simulink model "Ej_parcial_2019_sim"  (R2018a)
settings: Solver=FixedStepAuto  StartTime=0.0  StopTime=20  FixedStep=1e-5  RelTol=1e-3
values from neighbouring files (symbols this model uses):
  Ts = 0.0001    [Bolita_2.m]    (also in Ej_parcial_2019.m = 0.1; les_boles_de_les_pibardes.m = 0.01)
undefined symbols (not defined in the file or in its folder): DiscIntNeverNeededParam
settings Model: Creator=Guido L  LastModifiedBy=Guido L

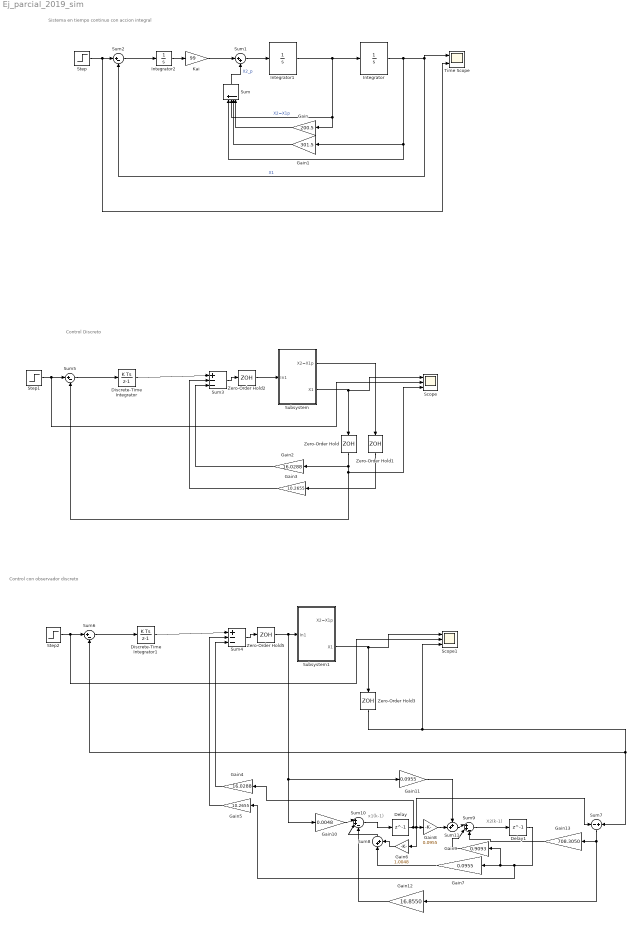
== system Ej_parcial_2019_sim ==
  note: X2(k-1)
  note: x1(k-1)
  note: Control con observador discreto
  note: Control Discreto
  note: Sistema en tiempo continuo con accion integral
  Delay : Delay  DelayLength=1
  Delay1 : Delay  DelayLength=1
  Discrete-Time Integrator : DiscreteIntegrator  gainval=3.8622  SampleTime=Ts  ICPrevOutput=DiscIntNeverNeededParam  ICPrevScaledInput=DiscIntNeverNeededParam
  Discrete-Time Integrator1 : DiscreteIntegrator  gainval=3.8622  SampleTime=Ts  ICPrevOutput=DiscIntNeverNeededParam  ICPrevScaledInput=DiscIntNeverNeededParam
  Gain : Gain  Gain=200.5
  Gain1 : Gain  Gain=301.5
  Gain10 : Gain  Gain=0.0048
  Gain11 : Gain  Gain=0.0955
  Gain12 : Gain  Gain=16.8550
  Gain13 : Gain  Gain=708.3050
  Gain2 : Gain  Gain=16.0288
  Gain3 : Gain  Gain=10.2655
  Gain4 : Gain  Gain=16.0288
  Gain5 : Gain  Gain=10.2655
  Gain6 : Gain  Gain=1.0048
  Gain7 : Gain  Gain=0.0955
  Gain8 : Gain  Gain=0.0955
  Gain9 : Gain  Gain=0.9093
  Integrator : Integrator
  Integrator1 : Integrator
  Integrator2 : Integrator
  Kai : Gain  Gain=99
  Scope : Scope  NumInputPorts=3
  Scope1 : Scope  NumInputPorts=3
  Step : Step  SampleTime=0
  Step1 : Step  SampleTime=1e-3
  Step2 : Step  SampleTime=1e-3
  Subsystem : Subsystem
  Subsystem1 : Subsystem
  Sum : Sum  Inputs=|+---
  Sum1 : Sum  Inputs=|++
  Sum10 : Sum  Inputs=|++-
  Sum11 : Sum  Inputs=++|
  Sum2 : Sum  Inputs=|+-
  Sum3 : Sum  Inputs=|+--
  Sum4 : Sum  Inputs=|+--
  Sum5 : Sum  Inputs=|+-
  Sum6 : Sum  Inputs=|+-
  Sum7 : Sum  Inputs=-|+
  Sum8 : Sum  Inputs=|++
  Sum9 : Sum  Inputs=|++-
  Time Scope : Scope  NumInputPorts=2
  Zero-Order Hold{,1..3,5} (5 alike) : ZeroOrderHold  SampleTime=Ts
  wires:
  Integrator/1 -> Gain1/1, Sum/1, Sum2/2, Time Scope/1  "X1"
  Integrator1/1 -> Sum/2, Gain/1, Integrator/1  "X2=X1p"
  Sum/1 -> Sum1/2  "X2_p"
  Sum1/1 -> Integrator1/1
  Kai/1 -> Sum1/1
  Integrator2/1 -> Kai/1
  Gain/1 -> Sum/4
  Gain1/1 -> Sum/3
  Sum2/1 -> Integrator2/1
  Step/1 -> Time Scope/2, Sum2/1
  Sum5/1 -> Discrete-Time Integrator/1
  Step1/1 -> Scope/2, Sum5/1
  Subsystem/2(X1) -> Scope/1, Zero-Order Hold/1
  Subsystem/1(X2=X1p) -> Zero-Order Hold1/1
  Zero-Order Hold/1 -> Scope/3, Sum5/2, Gain2/1
  Zero-Order Hold1/1 -> Gain3/1
  Zero-Order Hold2/1 -> Subsystem/1(In1)
  Discrete-Time Integrator/1 -> Sum3/1
  Sum3/1 -> Zero-Order Hold2/1
  Gain3/1 -> Sum3/2
  Gain2/1 -> Sum3/3
  Gain5/1 -> Sum4/2
  Sum4/1 -> Zero-Order Hold5/1
  Gain4/1 -> Sum4/3
  Discrete-Time Integrator1/1 -> Sum4/1
  Zero-Order Hold5/1 -> Gain11/1, Gain10/1, Subsystem1/1(In1)
  Step2/1 -> Scope1/2, Sum6/1
  Sum6/1 -> Discrete-Time Integrator1/1
  Subsystem1/2(X1) -> Scope1/1, Zero-Order Hold3/1
  Zero-Order Hold3/1 -> Sum6/2, Sum7/2, Scope1/3
  Delay/1 -> Gain4/1, Sum7/1, Gain6/1, Gain8/1
  Sum9/1 -> Delay1/1
  Delay1/1 -> Gain5/1, Gain9/1, Gain7/1
  Gain7/1 -> Sum8/1
  Gain6/1 -> Sum8/2
  Gain9/1 -> Sum9/2
  Gain10/1 -> Sum10/1
  Sum8/1 -> Sum10/2
  Sum10/1 -> Delay/1
  Sum11/1 -> Sum9/1
  Gain11/1 -> Sum11/1
  Gain8/1 -> Sum11/2
  Sum7/1 -> Gain13/1, Gain12/1
  Gain12/1 -> Sum10/3
  Gain13/1 -> Sum9/3

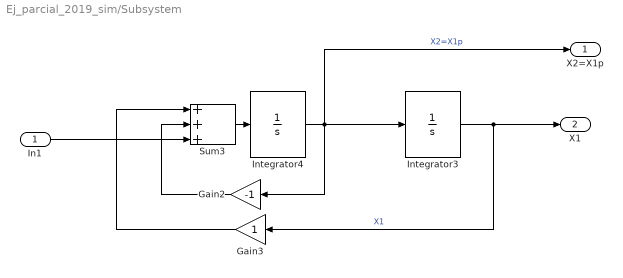
== system Ej_parcial_2019_sim/Subsystem ==
  In1 : Inport
  Gain2 : Gain  Gain=-1
  Gain3 : Gain
  Integrator3 : Integrator
  Integrator4 : Integrator
  Sum3 : Sum  Inputs=+++
  X2=X1p : Outport
  X1 : Outport  Port=2
  wires:
  Integrator4/1 -> X2=X1p/1, Gain2/1, Integrator3/1  "X2=X1p"
  In1/1 -> Sum3/3
  Integrator3/1 -> X1/1, Gain3/1  "X1"
  Gain2/1 -> Sum3/2
  Gain3/1 -> Sum3/1
  Sum3/1 -> Integrator4/1

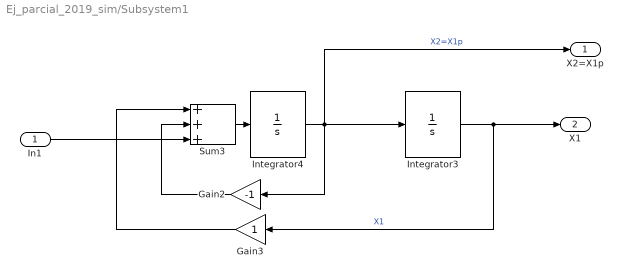
== system Ej_parcial_2019_sim/Subsystem1 ==
  In1 : Inport
  Gain2 : Gain  Gain=-1
  Gain3 : Gain
  Integrator3 : Integrator
  Integrator4 : Integrator
  Sum3 : Sum  Inputs=+++
  X2=X1p : Outport
  X1 : Outport  Port=2
  wires:
  Integrator4/1 -> X2=X1p/1, Gain2/1, Integrator3/1  "X2=X1p"
  In1/1 -> Sum3/3
  Integrator3/1 -> X1/1, Gain3/1  "X1"
  Gain2/1 -> Sum3/2
  Gain3/1 -> Sum3/1
  Sum3/1 -> Integrator4/1
